simulink model "differentiator_sFunc"  (R2021b)
settings: Solver=FixedStepDiscrete  StartTime=0.0  StopTime=20  FixedStep=0.01  RelTol=1e-3  EnableMultiTasking=on
model workspace (MAT data in the model file):
  enabled_mu = 'off'
  maskObj : Simulink.Mask (value not decoded)
  val_d = -1
  val_m = 2
libraries: simulink x4
settings Model: Creator=markusr  LastModifiedBy=matlabuser2
settings SolverCC: AlgebraicLoopSolver=TrustRegion
settings DataIOCC: LimitDataPoints=on  SaveFormat=Array  ReturnWorkspaceOutputs=off
settings OptimizationCC: LifeSpan=inf
settings DebuggingCC: UnderspecifiedInitializationDetection=Classic  MergeDetectMultiDrivingBlocksExec=none  SolverPrmCheckMsg=warning  SFUnexpectedBacktrackingDiag=warning  SFNoUnconditionalDefaultTransitionDiag=warning  SFExecutionAtInitializationDiag=none  SFMachineParentedDataDiag=warning  ArithmeticOperatorsInVariantConditions=warning
settings HardwareCC: ProdBitPerPointer=32  ProdBitPerSizeT=32  ProdBitPerPtrDiffT=32  ProdLargestAtomicFloat=None  ProdIntDivRoundTo=Undefined  ProdEndianess=Unspecified  ProdWordSize=32  ProdHWDeviceType=32-bit Generic
settings ModelReferenceCC: PropagateSignalLabelsOutOfModel=off
settings SFSimCC: SimUseLocalCustomCode=off  CustomCodeUndefinedFunction=UseInterfaceOnly
settings RTWCC: RTWUseLocalCustomCode=off
settings CodeAppCC: StateflowObjectComments=on
settings GRTTargetCC: TargetLangStandard=C89/C90 (ANSI)
settings ConfigComp: CovMetricSettings=dw  CovSaveCumulativeToWorkspaceVar=on  CovSaveSingleToWorkspaceVar=on  CovExternalEMLEnable=off

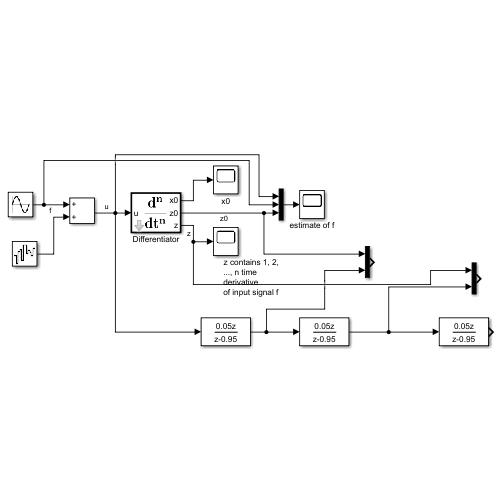
[thumbnail: Simulink's stored preview of the top-level diagram]
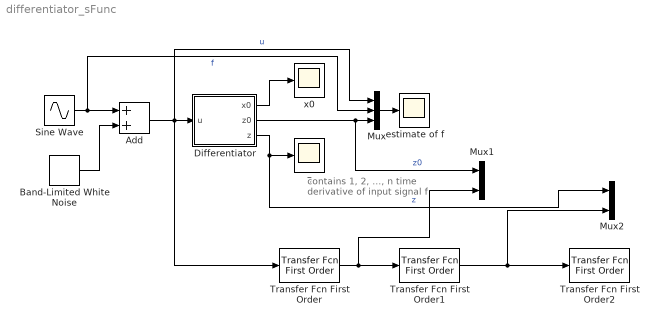
== system differentiator_sFunc ==
  note: contains 1, 2, ..., n time derivative
      | of input signal f
  Add : Sum
  Band-Limited White Noise : simulink/Sources/Band-Limited White Noise  Cov=[0.0001]  Ts=0.01  seed=[23341]
  Differentiator : Subsystem  TreatAsAtomicUnit=on  mask{n=2, r=1, Ts=0.01, filtering=on, nf=1, differentiator_type=Set Homogeneity Degree manually, d=-1, m=1, mu=1}
      mask prompts: n "n ="; r "r ="; Ts "Ts ="; filtering "Enable Filtering"; nf "nf ="; differentiator_type "Type of Differentiator"; d "d ="; m "m ="; mu "mu ="
      mask Callback filtering:
      | zzzzzzzzzz_maskObj = Simulink.Mask.get(gcb);
      | 
      | zzzzzzzzzz_enabled = get_param(gcb, 'filtering');
      | 
      | zzzzzzzzzz_nf_group = zzzzzzzzzz_maskObj.getDialogControl('nf_group');
      | zzzzzzzzzz_nf_group.DialogControls(3).Visible = zzzzzzzzzz_enabled;
      | zzzzzzzzzz_maskVisibilities = get_param(gcb,'maskVisibilities');
      | zzzzzzzzzz_maskVisibilities{5} = zzzzzzzzzz_enabled;
      | set_param(gcb,'maskVisibilities', zzzzzzzzzz_maskVisibilities);
      | if(strcmp(zzzzzzzzzz_enabled, 'off') == 1)
      |     set_param(gcb, 'nf', '0');
      | end
      | 
      | clear zzzzzzzzzz_nf_group zzzzzzzzzz_enabled zzzzzzzzzz_maskVisibilities zzzzzzzzzz_maskObj;
      mask TypeOptions differentiator_type: Linear Differentiator | Robust Exact Differentiator | Uniform Robust Exact Differentiator | Set Homogeneity Degree manually
      mask Callback differentiator_type:
      | zzzzzzzzzz_maskObj = Simulink.Mask.get(gcb);
      | 
      | zzzzzzzzzz_diff_type = get_param(gcb, 'differentiator_type');
      | zzzzzzzzzz_enabled_m = 'on';
      | zzzzzzzzzz_enabled = 'on';
      | zzzzzzzzzz_enabled_m2 = 'off';
      | zzzzzzzzzz_enabled_m3 = 'off';
      | 
      | zzzzzzzzzz_val_m = str2double(get_param(gcb, 'm'));
      | 
      | if(strcmp(zzzzzzzzzz_diff_type, 'Set Homogeneity Degree manually') == 1)
      |     zzzzzzzzzz_enabled_m3 = 'on';
      | else
      |     zzzzzzzzzz_enabled = 'off';
      |     if(strcmp(zzzzzzzzzz_diff_type, 'Linear Differentiator') == 1)
      |         set_param(gcb, 'd', '0');
      |         if(zzzzzzzzzz_val_m == 2)
      |             set_param(gcb, 'm', '1');
      |         end
      |     elseif(strcmp(zzzzzzzzzz_diff_type, 'Robust Exact Differentiator') == 1)
      |         zzzzzzzzzz_enabled_m2 = 'on';
      | 
      |         set_param(gcb, 'd', '-1');
      |     elseif(strcmp(zzzzzzzzzz_diff_type, 'Uniform Robust Exact Differentiator') == 1)
      |         set_param(gcb, 'd', '-1');
      |         set_param(gcb, 'm', '2');
      | 
      |         zzzzzzzzzz_enabled_m = 'off';
      |     end
      | end
      | 
      | zzzzzzzzzz_d_group = zzzzzzzzzz_maskObj.getDialogControl('d_group');
      | zzzzzzzzzz_d_group.DialogControls(2).Visible = zzzzzzzzzz_enabled;
      | zzzzzzzzzz_maskVisibilities = get_param(gcb,'maskVisibilities');
      | zzzzzzzzzz_maskVisibilities{7} = zzzzzzzzzz_enabled;
      | 
      | zzzzzzzzzz_m_group = zzzzzzzzzz_maskObj.getDialogControl('m_group');
      | zzzzzzzzzz_m_group.Visible = zzzzzzzzzz_enabled_m;
      | zzzzzzzzzz_m_group.DialogControls(2).Visible = zzzzzzzzzz_enabled_m2;
      | zzzzzzzzzz_m_group.DialogControls(3).Visible = zzzzzzzzzz_enabled_m3;
      | set_param(gcb,'maskVisibilities', zzzzzzzzzz_maskVisibilities);
      | 
      | clear zzzzzzzzzz_d_group zzzzzzzzzz_maskVisibilities zzzzzzzzzz_m_group zzzzzzzzzz_enabled_m;
      | clear zzzzzzzzzz_enabled_m2 zzzzzzzzzz_enabled_m3 zzzzzzzzzz_enabled zzzzzzzzzz_diff_type;
      | clear zzzzzzzzzz_val_m;
      | 
      | 
      | 
      | zzzzzzzzzz_val_m = str2double(get_param(gcb, 'm'));
      | zzzzzzzzzz_val_d = str2double(get_param(gcb, 'd'));
      | zzzzzzzzzz_enabled_mu = 'off';
      | if((isnan(zzzzzzzzzz_val_m) || zzzzzzzzzz_val_m == 2) && (isnan(zzzzzzzzzz_val_d) || zzzzzzzzzz_val_d == -1))
      |     zzzzzzzzzz_enabled_mu = 'on';
      | end
      | zzzzzzzzzz_maskObj.getDialogControl('mu_group').Visible = zzzzzzzzzz_enabled_mu;
      | clear zzzzzzzzzz_val_m zzzzzzzzzz_val_d zzzzzzzzzz_enabled_mu zzzzzzzzzz_maskObj;
      | clear zzzzzzzzzz_maskObj
      mask Callback d:
      | zzzzzzzzzz_maskObj = Simulink.Mask.get(gcb);
      | zzzzzzzzzz_val_m = str2double(get_param(gcb, 'm'));
      | zzzzzzzzzz_val_d = str2double(get_param(gcb, 'd'));
      | zzzzzzzzzz_enabled_mu = 'off';
      | if((isnan(zzzzzzzzzz_val_m) || zzzzzzzzzz_val_m == 2) && (isnan(zzzzzzzzzz_val_d) || zzzzzzzzzz_val_d == -1))
      |     zzzzzzzzzz_enabled_mu = 'on';
      | end
      | zzzzzzzzzz_maskObj.getDialogControl('mu_group').Visible = zzzzzzzzzz_enabled_mu;
      | clear zzzzzzzzzz_val_m zzzzzzzzzz_val_d zzzzzzzzzz_enabled_mu zzzzzzzzzz_maskObj;
      | clear zzzzzzzzzz_maskObj
      mask Callback m:
      | zzzzzzzzzz_maskObj = Simulink.Mask.get(gcb);
      | zzzzzzzzzz_val_m = str2double(get_param(gcb, 'm'));
      | zzzzzzzzzz_val_d = str2double(get_param(gcb, 'd'));
      | zzzzzzzzzz_enabled_mu = 'off';
      | if((isnan(zzzzzzzzzz_val_m) || zzzzzzzzzz_val_m == 2) && (isnan(zzzzzzzzzz_val_d) || zzzzzzzzzz_val_d == -1))
      |     zzzzzzzzzz_enabled_mu = 'on';
      | end
      | zzzzzzzzzz_maskObj.getDialogControl('mu_group').Visible = zzzzzzzzzz_enabled_mu;
      | clear zzzzzzzzzz_val_m zzzzzzzzzz_val_d zzzzzzzzzz_enabled_mu zzzzzzzzzz_maskObj;
      | clear zzzzzzzzzz_maskObj
      mask DialogControl DescGroupVar Prompt: Differentiator Toolbox v3
      mask DialogControl DescTextVar Prompt: This block provides estimates of the derivatives of the input signal.
      mask DialogControl DescTextVar_2 Prompt: The first scalar output x0 provides a convergence measure. Increase the robustness factor 'r' to ensure that this signal converges to a sufficiently small neighborhood of zero.
      mask DialogControl DescTextVar_3 Prompt: The second output z0 is an estimate of the input signal.
      mask DialogControl DescTextVar_4 Prompt: The third output z is a vector containing the estimated derivatives of the input signal. The length of this vector equals the chosen differentiaton order 'n'.
      mask DialogControl DescTextVar_5 Prompt: The sum of 'n' (differentiation order) and 'nf' (filtering order) must not exceed 10.
      mask DialogControl n_group Prompt: Differentiation Order
      mask DialogControl n_desc Prompt: Number of derivatives to be estimated for input signal.
      mask DialogControl r_group Prompt: Robustness Factor
      mask DialogControl r_desc Prompt: Set r to a positive value. This value is proportional to the continuous time closed loop eigenvalues.
      mask DialogControl Ts_group Prompt: Step size
      mask DialogControl Ts_desc Prompt: Simulation Sample Time (-1 for inherited).
      mask DialogControl Advanced Prompt: Advanced Options
      mask DialogControl nf_group Prompt: Filter Options
      mask DialogControl DescTextVar_copy Prompt: Use the filtering option, if there is noise present. Adjust the Filtering Order 'nf' to achieve better estimations for the derivatives. Usually, a filtering order of 1 or 2 is sufficient.
      mask DialogControl nf_desc Prompt: Filtering Order.
      mask DialogControl d_group Prompt: Differentiator Options
      mask DialogControl d_desc Prompt: Set the homogeneity degree to a value between -1 (Robust Exact Differentiator) and 0 (Linear Differentiator).
      mask DialogControl m_group Prompt: Discretization Method
      mask DialogControl m_desc Prompt: Select m out of {0, 1}, where 0 corresponds to Forward Euler eigenvalue mapping and 1 corresponds to Matching Approach.
      mask DialogControl m_desc_copy Prompt: Set m to 2 for Uniform Robust Exact Differentiator behavior.
      mask DialogControl m_desc_copy_copy Prompt: Set m to 2 for Uniform Robust Exact Differentiator behavior (only available for d=-1).
      mask DialogControl mu_group Prompt: Eigenvalue tuning gain for Uniform RED
      mask DialogControl mu_desc Prompt: Set mu to a positive value. mu is a tuning gain for the eigenvalue selection of the Uniform Robust Exact Differentiator.
      mask Display:
      | image('image.png');
      | port_label('input', 1, 'u')
      | port_label('output', 1, 'x0')
      | port_label('output', 2, 'z0')
      | port_label('output', 3, 'z')
  Mux : Mux  Inputs=3
  Mux1 : Mux  Inputs=2
  Mux2 : Mux  Inputs=2
  Sine Wave : Sin  Bias=2
  Transfer Fcn First Order : simulink/Discrete/Transfer Fcn First Order  PoleZ=0.95  ICPrevOutput=0.0  DoSatur=off
  Transfer Fcn First Order1 : simulink/Discrete/Transfer Fcn First Order  PoleZ=0.95  ICPrevOutput=0.0  DoSatur=off
  Transfer Fcn First Order2 : simulink/Discrete/Transfer Fcn First Order  PoleZ=0.95  ICPrevOutput=0.0  DoSatur=off
  estimate of f : Scope
  x0 : Scope
  z : Scope
  wires:
  Differentiator/1(x0) -> x0/1
  Differentiator/3(z) -> Mux2/1, z/1  "z"
  Mux/1 -> estimate of f/1
  Sine Wave/1 -> Add/1, Mux/2  "f"
  Add/1 -> Transfer Fcn First Order/1, Differentiator/1(u), Mux/1  "u"
  Differentiator/2(z0) -> Mux1/1, Mux/3  "z0"
  Band-Limited White Noise/1 -> Add/2
  Transfer Fcn First Order/1 -> Mux1/2, Transfer Fcn First Order1/1
  Transfer Fcn First Order1/1 -> Transfer Fcn First Order2/1, Mux2/2

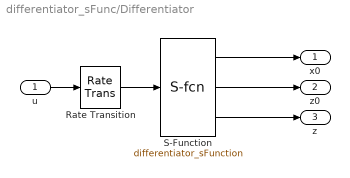
== system differentiator_sFunc/Differentiator ==
  u : Inport
  Rate Transition : RateTransition
  S-Function : S-Function  FunctionName=differentiator_sFunction  Parameters=n,nf,d,r,m,mu,Ts  SFunctionDeploymentMode=off  EnableBusSupport=off
  x0 : Outport  VectorParamsAs1DForOutWhenUnconnected=off
  z0 : Outport  Port=2  VectorParamsAs1DForOutWhenUnconnected=off
  z : Outport  Port=3  VectorParamsAs1DForOutWhenUnconnected=off
  wires:
  S-Function/3 -> z/1
  S-Function/1 -> x0/1
  S-Function/2 -> z0/1
  u/1 -> Rate Transition/1
  Rate Transition/1 -> S-Function/1
